simulink model "simple_puma560controller"  (R2020a)
settings: Solver=VariableStepAuto  StartTime=0.0  StopTime=5  RelTol=1e-3
libraries: roblocks x3
settings Model: Creator=yrza  LastModifiedBy=Kasumi

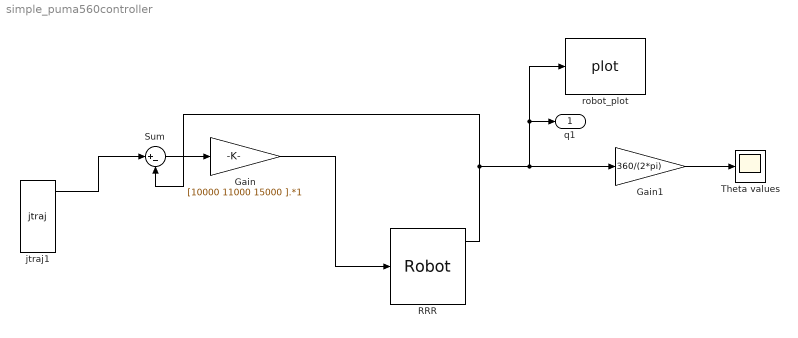
== system simple_puma560controller ==
  Gain : Gain  Gain=[10000 11000 15000 ].*1
  Gain1 : Gain  Gain=360/(2*pi)
  RRR : roblocks/Arm/Robot  robot=RRR  q0=[0 0 0]
  Sum : Sum  Inputs=|+-
  Theta values : Scope
  jtraj1 : roblocks/Toolbox/jtraj  q0=[0 0 0]  qf=[pi/2 -pi/4 -pi/4]  tmax=2  ts=0.02
  robot_plot : roblocks/Arm/plot  robot=RRR  fps=5  holdplot=on
  q1 : Outport
  wires:
  RRR/1 -> robot_plot/1, q1/1, Gain1/1, Sum/2
  Gain1/1 -> Theta values/1
  jtraj1/1 -> Sum/1
  Gain/1 -> RRR/1
  Sum/1 -> Gain/1
